simulink library "newTires"  (R2019b)
settings: Solver=ode45  StartTime=0.0  StopTime=10.0  RelTol=1e-3  EnableMultiTasking=on
libraries: vehdynlibtirecommon x6, autolibshared x4, autolibsharedcommon x1
(part 3 of 3)

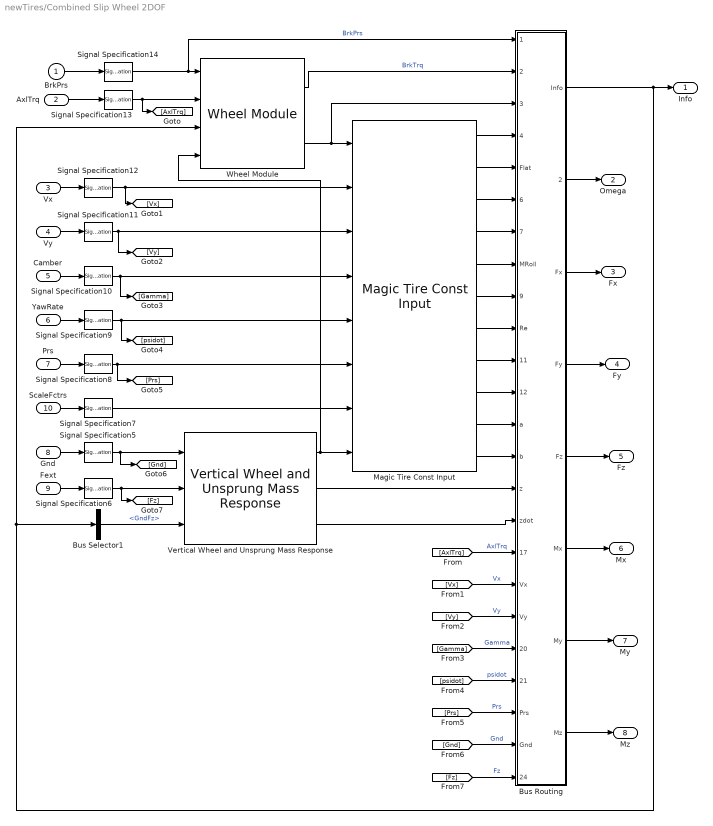
== system newTires/Combined Slip Wheel 2DOF ==
  BrkPrs : Inport
  AxlTrq : Inport  Port=2
  Vx : Inport  Port=3
  Vy : Inport  Port=4
  Camber : Inport  Port=5
  YawRate : Inport  Port=6
  Prs : Inport  Port=7
  Gnd : Inport  Port=8
  Fext : Inport  Port=9
  ScaleFctrs : Inport  Port=10
  Bus Selector1 : BusSelector  OutputSignals=GndFz
  Bus Routing : Subsystem
  Magic Tire Const Input : vehdynlibtirecommon/Magic Tire Const Input  SystemSampleTime=-1  Latency=0  AutoFrameSizeCalculation=off
      settings: SourceProductName=Vehicle Dynamics Blockset  SourceProductBaseCode=VE
  Signal Specification10 : SignalSpecification  Unit=rad
  Signal Specification11 : SignalSpecification  Unit=m/s
  Signal Specification12 : SignalSpecification  Unit=m/s
  Signal Specification13 : SignalSpecification  Unit=N*m
  Signal Specification14 : SignalSpecification  Unit=Pa
  Signal Specification5 : SignalSpecification  Unit=m
  Signal Specification6 : SignalSpecification  Unit=N
  Signal Specification7 : SignalSpecification  Unit=1
  Signal Specification8 : SignalSpecification  Unit=Pa
  Signal Specification9 : SignalSpecification  Unit=rad/s
  Vertical Wheel and Unsprung Mass Response : vehdynlibtirecommon/Vertical Wheel and Unsprung Mass Response  m=MASS  bz=VERTICAL_DAMPING  zo=zo  zdoto=zdoto  g=GRAVITY  ReMax=UNLOADED_RADIUS
      settings: SourceProductName=Vehicle Dynamics Blockset  SourceProductBaseCode=VE
  Wheel Module : vehdynlibtirecommon/Wheel Module  Iyy=IYY
      settings: SourceProductName=Vehicle Dynamics Blockset  SourceProductBaseCode=VE
  Info : Outport  VectorParamsAs1DForOutWhenUnconnected=off
  Omega : Outport  Port=2  Unit=rad/s  VectorParamsAs1DForOutWhenUnconnected=off
  Fx : Outport  Port=3  Unit=N  VectorParamsAs1DForOutWhenUnconnected=off
  Fy : Outport  Port=4  Unit=N  VectorParamsAs1DForOutWhenUnconnected=off
  Fz : Outport  Port=5  Unit=N  VectorParamsAs1DForOutWhenUnconnected=off
  Mx : Outport  Port=6  Unit=N*m  VectorParamsAs1DForOutWhenUnconnected=off
  My : Outport  Port=7  Unit=N*m  VectorParamsAs1DForOutWhenUnconnected=off
  Mz : Outport  Port=8  Unit=N*m  VectorParamsAs1DForOutWhenUnconnected=off
  wires:
  Wheel Module/1 -> Bus Routing/2(BrkTrq)  "BrkTrq"
  Vertical Wheel and Unsprung Mass Response/1 -> Magic Tire Const Input/8, Wheel Module/4
  Wheel Module/2 -> Magic Tire Const Input/1, Bus Routing/3(omega)
  Signal Specification5/1 -> [Gnd], Vertical Wheel and Unsprung Mass Response/1
  Gnd/1 -> Signal Specification5/1
  Fext/1 -> Signal Specification6/1
  Signal Specification6/1 -> [Fz], Vertical Wheel and Unsprung Mass Response/2
  Signal Specification7/1 -> Magic Tire Const Input/7
  Prs/1 -> Signal Specification8/1
  Signal Specification8/1 -> [Prs], Magic Tire Const Input/6
  YawRate/1 -> Signal Specification9/1
  Signal Specification9/1 -> [psidot], Magic Tire Const Input/5
  ScaleFctrs/1 -> Signal Specification7/1
  Signal Specification10/1 -> [Gamma], Magic Tire Const Input/4
  Camber/1 -> Signal Specification10/1
  Signal Specification11/1 -> [Vy], Magic Tire Const Input/3
  Vy/1 -> Signal Specification11/1
  Vx/1 -> Signal Specification12/1
  Signal Specification12/1 -> [Vx], Magic Tire Const Input/2
  Signal Specification13/1 -> [AxlTrq], Wheel Module/2
  AxlTrq/1 -> Signal Specification13/1
  Signal Specification14/1 -> Bus Routing/1(BrkPrs), Wheel Module/1  "BrkPrs"
  Bus Selector1/1 -> Vertical Wheel and Unsprung Mass Response/3  "<GndFz>"
  BrkPrs/1 -> Signal Specification14/1
  Bus Routing/1(Info) -> Bus Selector1/1, Wheel Module/3, Info/1
  Magic Tire Const Input/1 -> Bus Routing/4(FLong)
  Magic Tire Const Input/2 -> Bus Routing/5(Flat)
  Magic Tire Const Input/3 -> Bus Routing/6(FzTire)
  Magic Tire Const Input/4 -> Bus Routing/7(MOver)
  Magic Tire Const Input/5 -> Bus Routing/8(MRoll)
  Magic Tire Const Input/6 -> Bus Routing/9(MAlign)
  Magic Tire Const Input/7 -> Bus Routing/10(Re)
  Magic Tire Const Input/8 -> Bus Routing/11(Kappa)
  Magic Tire Const Input/9 -> Bus Routing/12(Alpha)
  Magic Tire Const Input/10 -> Bus Routing/13(a)
  Magic Tire Const Input/11 -> Bus Routing/14(b)
  Vertical Wheel and Unsprung Mass Response/2 -> Bus Routing/15(z)
  Vertical Wheel and Unsprung Mass Response/3 -> Bus Routing/16(zdot)
  Bus Routing/2(Omega) -> Omega/1
  Bus Routing/3(Fx) -> Fx/1
  Bus Routing/4(Fy) -> Fy/1
  Bus Routing/5(Fz) -> Fz/1
  Bus Routing/6(Mx) -> Mx/1
  Bus Routing/7(My) -> My/1
  Bus Routing/8(Mz) -> Mz/1
  [AxlTrq] -> Bus Routing/17(AxlTrq)  "AxlTrq"
  [Vx] -> Bus Routing/18(Vx)  "Vx"
  [Vy] -> Bus Routing/19(Vy)  "Vy"
  [Gamma] -> Bus Routing/20(Gamma)  "Gamma"
  [psidot] -> Bus Routing/21(psidot)  "psidot"
  [Prs] -> Bus Routing/22(Prs)  "Prs"
  [Gnd] -> Bus Routing/23(Gnd)  "Gnd"
  [Fz] -> Bus Routing/24(FNormal)  "Fz"

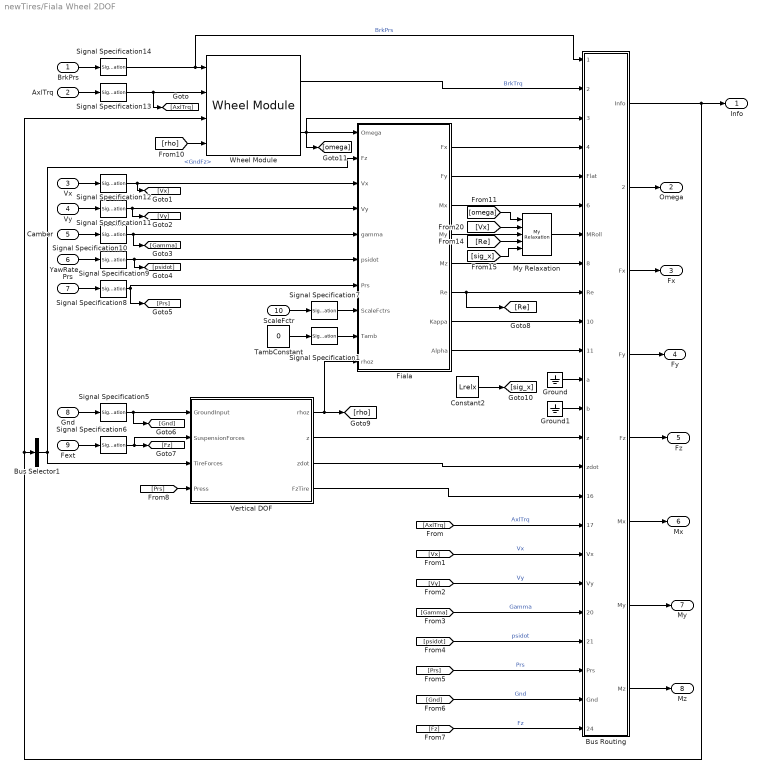
== system newTires/Fiala Wheel 2DOF ==
  BrkPrs : Inport
  AxlTrq : Inport  Port=2
  Vx : Inport  Port=3
  Vy : Inport  Port=4
  Camber : Inport  Port=5
  YawRate : Inport  Port=6
  Prs : Inport  Port=7
  Gnd : Inport  Port=8
  Fext : Inport  Port=9  Unit=N
  ScaleFctr : Inport  Port=10
  Bus Selector1 : BusSelector  OutputSignals=GndFz
  Bus Routing : Subsystem
  Constant2 : Constant  Value=Lrelx
  Fiala : Subsystem
  Ground : Ground
  Ground1 : Ground
  My Relaxation : vehdynlibtirecommon/Magic Tire Const Input/My Relaxation  UpperValue=.001
      settings: SourceProductName=Vehicle Dynamics Blockset  SourceProductBaseCode=VE
  Signal Specification1 : SignalSpecification  Unit=K
  Signal Specification10 : SignalSpecification  Unit=rad
  Signal Specification11 : SignalSpecification  Unit=m/s
  Signal Specification12 : SignalSpecification  Unit=m/s
  Signal Specification13 : SignalSpecification  Unit=N*m
  Signal Specification14 : SignalSpecification  Unit=Pa
  Signal Specification5 : SignalSpecification  Unit=m
  Signal Specification6 : SignalSpecification  Unit=N
  Signal Specification7 : SignalSpecification  Unit=1
  Signal Specification8 : SignalSpecification  Unit=Pa
  Signal Specification9 : SignalSpecification  Unit=rad/s
  TambConstant : Constant  Value=0
  Vertical DOF : Subsystem  VariantControlMode=Label  Variant=on  VariantControl=Variant1  LabelModeActiveChoice=None
  Wheel Module : vehdynlibtirecommon/Wheel Module  Iyy=IYY
      settings: SourceProductName=Vehicle Dynamics Blockset  SourceProductBaseCode=VE
  Info : Outport  VectorParamsAs1DForOutWhenUnconnected=off
  Omega : Outport  Port=2  Unit=rad/s  VectorParamsAs1DForOutWhenUnconnected=off
  Fx : Outport  Port=3  Unit=N  VectorParamsAs1DForOutWhenUnconnected=off
  Fy : Outport  Port=4  Unit=N  VectorParamsAs1DForOutWhenUnconnected=off
  Fz : Outport  Port=5  Unit=N  VectorParamsAs1DForOutWhenUnconnected=off
  Mx : Outport  Port=6  Unit=N*m  VectorParamsAs1DForOutWhenUnconnected=off
  My : Outport  Port=7  Unit=N*m  VectorParamsAs1DForOutWhenUnconnected=off
  Mz : Outport  Port=8  Unit=N*m  VectorParamsAs1DForOutWhenUnconnected=off
  wires:
  Constant2/1 -> [sig_x]
  Fiala/6(Re) -> [Re], Bus Routing/9(Re)
  [Re] -> My Relaxation/4
  [omega] -> My Relaxation/1
  [Vx] -> My Relaxation/2
  [sig_x] -> My Relaxation/5
  Wheel Module/1 -> Bus Routing/2(BrkTrq)  "BrkTrq"
  Wheel Module/2 -> Fiala/1(Omega), Bus Routing/3(omega), [omega]
  Signal Specification5/1 -> [Gnd], Vertical DOF/1("GroundInput ")
  Gnd/1 -> Signal Specification5/1
  Fext/1 -> Signal Specification6/1
  Signal Specification6/1 -> [Fz], Vertical DOF/2("SuspensionForces ")
  Signal Specification7/1 -> Fiala/8(ScaleFctrs)
  Prs/1 -> Signal Specification8/1
  Signal Specification8/1 -> Fiala/7(Prs), [Prs]
  YawRate/1 -> Signal Specification9/1
  Signal Specification9/1 -> Fiala/6(psidot), [psidot]
  ScaleFctr/1 -> Signal Specification7/1
  Signal Specification10/1 -> Fiala/5(gamma), [Gamma]
  Camber/1 -> Signal Specification10/1
  Signal Specification11/1 -> [Vy], Fiala/4(Vy)
  Vy/1 -> Signal Specification11/1
  Vx/1 -> Signal Specification12/1
  Signal Specification12/1 -> [Vx], Fiala/3(Vx)
  Signal Specification13/1 -> [AxlTrq], Wheel Module/2
  AxlTrq/1 -> Signal Specification13/1
  Signal Specification14/1 -> Bus Routing/1(BrkPrs), Wheel Module/1  "BrkPrs"
  Bus Selector1/1 -> Fiala/2(Fz), Vertical DOF/3("TireForces ")  "<GndFz>"
  Bus Routing/1(Info) -> Bus Selector1/1, Wheel Module/3, Info/1
  Fiala/5(Mz) -> Bus Routing/8(MAlign)
  Fiala/7(Kappa) -> Bus Routing/10(Kappa)
  Fiala/8(Alpha) -> Bus Routing/11(Alpha)
  Ground/1 -> Bus Routing/12(a)
  Ground1/1 -> Bus Routing/13(b)
  Bus Routing/2(Omega) -> Omega/1
  Bus Routing/3(Fx) -> Fx/1
  Bus Routing/4(Fy) -> Fy/1
  Bus Routing/5(Fz) -> Fz/1
  Bus Routing/6(Mx) -> Mx/1
  Bus Routing/7(My) -> My/1
  Bus Routing/8(Mz) -> Mz/1
  [AxlTrq] -> Bus Routing/17(AxlTrq)  "AxlTrq"
  [Vx] -> Bus Routing/18(Vx)  "Vx"
  [Vy] -> Bus Routing/19(Vy)  "Vy"
  [Gamma] -> Bus Routing/20(Gamma)  "Gamma"
  [psidot] -> Bus Routing/21(psidot)  "psidot"
  [Prs] -> Bus Routing/22(Prs)  "Prs"
  [Gnd] -> Bus Routing/23(Gnd)  "Gnd"
  [Fz] -> Bus Routing/24(FNormal)  "Fz"
  Fiala/3(Mx) -> Bus Routing/6(MOver)
  Fiala/2(Fy) -> Bus Routing/5(Flat)
  Fiala/1(Fx) -> Bus Routing/4(FLong)
  Fiala/4(My) -> My Relaxation/3
  My Relaxation/1 -> Bus Routing/7(MRoll)
  [rho] -> Wheel Module/4
  BrkPrs/1 -> Signal Specification14/1
  Signal Specification1/1 -> Fiala/9(Tamb)
  Vertical DOF/1(" rhoz") -> Fiala/10(rhoz), [rho]
  Vertical DOF/2(" z") -> Bus Routing/14(z)
  Vertical DOF/3(" zdot") -> Bus Routing/15(zdot)
  [Prs] -> Vertical DOF/4(Press)
  TambConstant/1 -> Signal Specification1/1
  Vertical DOF/4(FzTire) -> Bus Routing/16(GndFz)

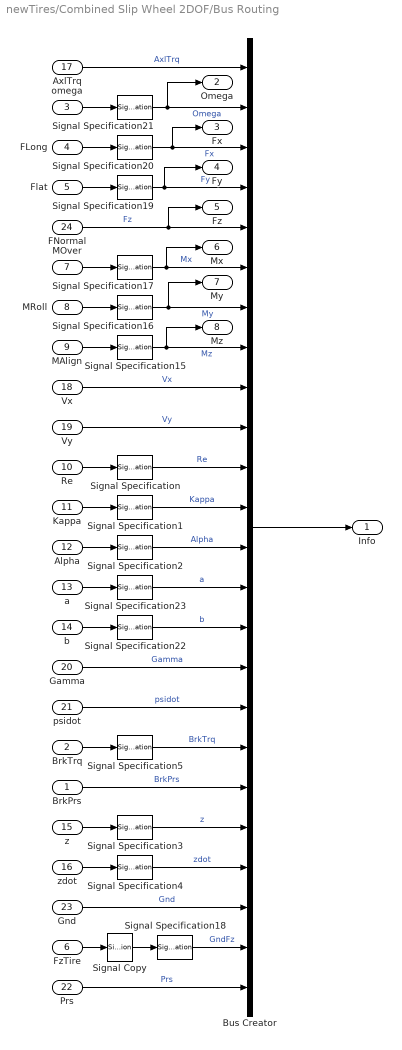
== system newTires/Combined Slip Wheel 2DOF/Bus Routing ==
  BrkPrs : Inport
  BrkTrq : Inport  Port=2
  omega : Inport  Port=3
  FLong : Inport  Port=4
  Flat : Inport  Port=5
  FzTire : Inport  Port=6
  MOver : Inport  Port=7
  MRoll : Inport  Port=8
  MAlign : Inport  Port=9
  Re : Inport  Port=10
  Kappa : Inport  Port=11
  Alpha : Inport  Port=12
  a : Inport  Port=13
  b : Inport  Port=14
  z : Inport  Port=15
  zdot : Inport  Port=16
  AxlTrq : Inport  Port=17
  Vx : Inport  Port=18
  Vy : Inport  Port=19
  Gamma : Inport  Port=20
  psidot : Inport  Port=21
  Prs : Inport  Port=22
  Gnd : Inport  Port=23
  FNormal : Inport  Port=24
  Bus Creator : BusCreator  Inputs=24
  Signal Copy : SignalConversion  OverrideOpt=off
  Signal Specification{,3,22..23} (4 alike) : SignalSpecification  Unit=m
  Signal Specification1 : SignalSpecification  Unit=1
  Signal Specification{5,15..17} (4 alike) : SignalSpecification  Unit=N*m
  Signal Specification18 : SignalSpecification  Unit=N
  Signal Specification19 : SignalSpecification  Unit=N
  Signal Specification2 : SignalSpecification  Unit=rad
  Signal Specification20 : SignalSpecification  Unit=N
  Signal Specification21 : SignalSpecification  Unit=rad/s
  Signal Specification4 : SignalSpecification  Unit=m/s
  Info : Outport  VectorParamsAs1DForOutWhenUnconnected=off
  Omega : Outport  Port=2  Unit=rad/s  VectorParamsAs1DForOutWhenUnconnected=off
  Fx : Outport  Port=3  Unit=N  VectorParamsAs1DForOutWhenUnconnected=off
  Fy : Outport  Port=4  Unit=N  VectorParamsAs1DForOutWhenUnconnected=off
  Fz : Outport  Port=5  Unit=N  VectorParamsAs1DForOutWhenUnconnected=off
  Mx : Outport  Port=6  Unit=N*m  VectorParamsAs1DForOutWhenUnconnected=off
  My : Outport  Port=7  Unit=N*m  VectorParamsAs1DForOutWhenUnconnected=off
  Mz : Outport  Port=8  Unit=N*m  VectorParamsAs1DForOutWhenUnconnected=off
  wires:
  Signal Specification3/1 -> Bus Creator/20  "z"
  a/1 -> Signal Specification23/1
  Alpha/1 -> Signal Specification2/1
  Signal Specification4/1 -> Bus Creator/21  "zdot"
  Signal Specification21/1 -> Bus Creator/2, Omega/1  "Omega"
  FNormal/1 -> Bus Creator/5, Fz/1  "Fz"
  Signal Specification15/1 -> Bus Creator/8, Mz/1  "Mz"
  Signal Specification/1 -> Bus Creator/11  "Re"
  Bus Creator/1 -> Info/1
  Signal Specification17/1 -> Mx/1, Bus Creator/6  "Mx"
  MOver/1 -> Signal Specification17/1
  Signal Specification1/1 -> Bus Creator/12  "Kappa"
  FLong/1 -> Signal Specification20/1
  Signal Specification19/1 -> Bus Creator/4, Fy/1  "Fy"
  Signal Specification16/1 -> Bus Creator/7, My/1  "My"
  omega/1 -> Signal Specification21/1
  Signal Specification2/1 -> Bus Creator/13  "Alpha"
  Signal Specification20/1 -> Bus Creator/3, Fx/1  "Fx"
  Signal Specification23/1 -> Bus Creator/14  "a"
  Signal Specification22/1 -> Bus Creator/15  "b"
  FzTire/1 -> Signal Copy/1
  MAlign/1 -> Signal Specification15/1
  Flat/1 -> Signal Specification19/1
  b/1 -> Signal Specification22/1
  Re/1 -> Signal Specification/1
  zdot/1 -> Signal Specification4/1
  z/1 -> Signal Specification3/1
  MRoll/1 -> Signal Specification16/1
  Kappa/1 -> Signal Specification1/1
  BrkTrq/1 -> Signal Specification5/1
  AxlTrq/1 -> Bus Creator/1  "AxlTrq"
  Vx/1 -> Bus Creator/9  "Vx"
  Vy/1 -> Bus Creator/10  "Vy"
  Gamma/1 -> Bus Creator/16  "Gamma"
  psidot/1 -> Bus Creator/17  "psidot"
  Signal Specification5/1 -> Bus Creator/18  "BrkTrq"
  BrkPrs/1 -> Bus Creator/19  "BrkPrs"
  Signal Specification18/1 -> Bus Creator/23  "GndFz"
  Gnd/1 -> Bus Creator/22  "Gnd"
  Prs/1 -> Bus Creator/24  "Prs"
  Signal Copy/1 -> Signal Specification18/1

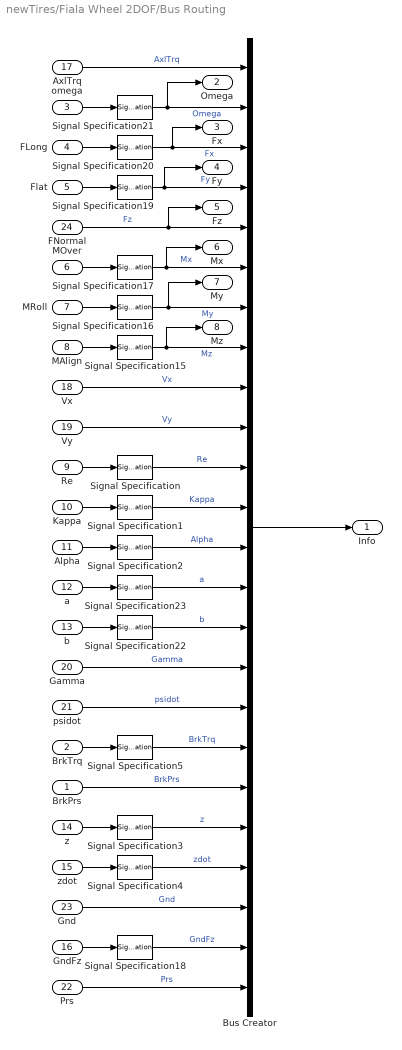
== system newTires/Fiala Wheel 2DOF/Bus Routing ==
  BrkPrs : Inport
  BrkTrq : Inport  Port=2
  omega : Inport  Port=3
  FLong : Inport  Port=4
  Flat : Inport  Port=5
  MOver : Inport  Port=6
  MRoll : Inport  Port=7
  MAlign : Inport  Port=8
  Re : Inport  Port=9
  Kappa : Inport  Port=10
  Alpha : Inport  Port=11
  a : Inport  Port=12
  b : Inport  Port=13
  z : Inport  Port=14
  zdot : Inport  Port=15
  GndFz : Inport  Port=16
  AxlTrq : Inport  Port=17
  Vx : Inport  Port=18
  Vy : Inport  Port=19
  Gamma : Inport  Port=20
  psidot : Inport  Port=21
  Prs : Inport  Port=22
  Gnd : Inport  Port=23
  FNormal : Inport  Port=24
  Bus Creator : BusCreator  Inputs=24
  Signal Specification{,3,22..23} (4 alike) : SignalSpecification  Unit=m
  Signal Specification1 : SignalSpecification  Unit=1
  Signal Specification{5,15..17} (4 alike) : SignalSpecification  Unit=N*m
  Signal Specification18 : SignalSpecification  Unit=N
  Signal Specification19 : SignalSpecification  Unit=N
  Signal Specification2 : SignalSpecification  Unit=rad
  Signal Specification20 : SignalSpecification  Unit=N
  Signal Specification21 : SignalSpecification  Unit=rad/s
  Signal Specification4 : SignalSpecification  Unit=m/s
  Info : Outport  VectorParamsAs1DForOutWhenUnconnected=off
  Omega : Outport  Port=2  Unit=rad/s  VectorParamsAs1DForOutWhenUnconnected=off
  Fx : Outport  Port=3  Unit=N  VectorParamsAs1DForOutWhenUnconnected=off
  Fy : Outport  Port=4  Unit=N  VectorParamsAs1DForOutWhenUnconnected=off
  Fz : Outport  Port=5  Unit=N  VectorParamsAs1DForOutWhenUnconnected=off
  Mx : Outport  Port=6  Unit=N*m  VectorParamsAs1DForOutWhenUnconnected=off
  My : Outport  Port=7  Unit=N*m  VectorParamsAs1DForOutWhenUnconnected=off
  Mz : Outport  Port=8  Unit=N*m  VectorParamsAs1DForOutWhenUnconnected=off
  wires:
  Signal Specification3/1 -> Bus Creator/20  "z"
  a/1 -> Signal Specification23/1
  Alpha/1 -> Signal Specification2/1
  Signal Specification4/1 -> Bus Creator/21  "zdot"
  Signal Specification21/1 -> Bus Creator/2, Omega/1  "Omega"
  FNormal/1 -> Bus Creator/5, Fz/1  "Fz"
  Signal Specification15/1 -> Bus Creator/8, Mz/1  "Mz"
  Signal Specification/1 -> Bus Creator/11  "Re"
  Bus Creator/1 -> Info/1
  Signal Specification17/1 -> Mx/1, Bus Creator/6  "Mx"
  MOver/1 -> Signal Specification17/1
  Signal Specification1/1 -> Bus Creator/12  "Kappa"
  FLong/1 -> Signal Specification20/1
  Signal Specification19/1 -> Bus Creator/4, Fy/1  "Fy"
  Signal Specification16/1 -> Bus Creator/7, My/1  "My"
  omega/1 -> Signal Specification21/1
  Signal Specification2/1 -> Bus Creator/13  "Alpha"
  Signal Specification20/1 -> Bus Creator/3, Fx/1  "Fx"
  Signal Specification23/1 -> Bus Creator/14  "a"
  Signal Specification22/1 -> Bus Creator/15  "b"
  GndFz/1 -> Signal Specification18/1
  MAlign/1 -> Signal Specification15/1
  Flat/1 -> Signal Specification19/1
  b/1 -> Signal Specification22/1
  Re/1 -> Signal Specification/1
  zdot/1 -> Signal Specification4/1
  z/1 -> Signal Specification3/1
  MRoll/1 -> Signal Specification16/1
  Kappa/1 -> Signal Specification1/1
  BrkTrq/1 -> Signal Specification5/1
  AxlTrq/1 -> Bus Creator/1  "AxlTrq"
  Vx/1 -> Bus Creator/9  "Vx"
  Vy/1 -> Bus Creator/10  "Vy"
  Gamma/1 -> Bus Creator/16  "Gamma"
  psidot/1 -> Bus Creator/17  "psidot"
  Signal Specification5/1 -> Bus Creator/18  "BrkTrq"
  BrkPrs/1 -> Bus Creator/19  "BrkPrs"
  Signal Specification18/1 -> Bus Creator/23  "GndFz"
  Gnd/1 -> Bus Creator/22  "Gnd"
  Prs/1 -> Bus Creator/24  "Prs"

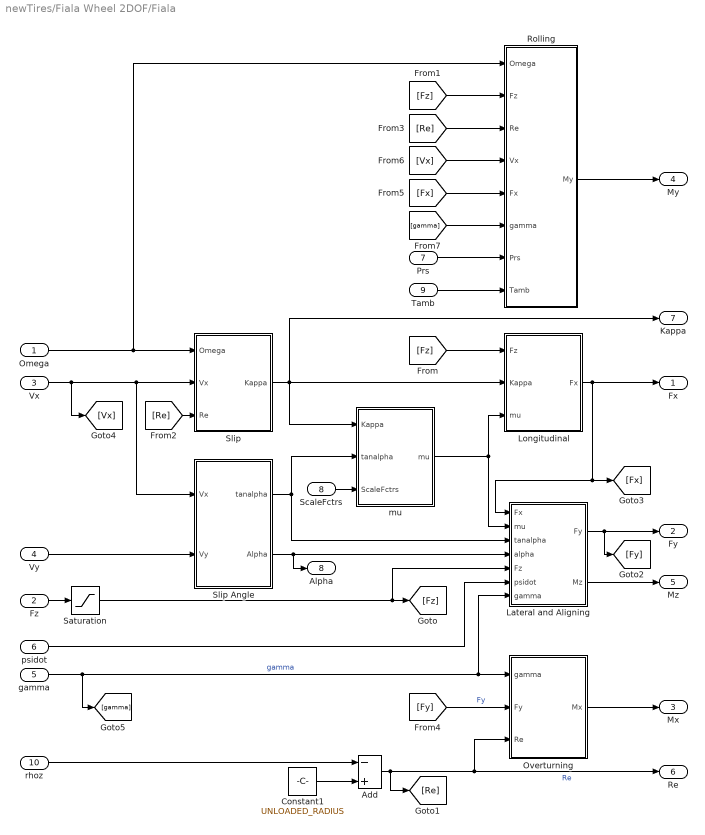
== system newTires/Fiala Wheel 2DOF/Fiala ==
  Omega : Inport
  Fz : Inport  Port=2
  Vx : Inport  Port=3
  Vy : Inport  Port=4
  gamma : Inport  Port=5
  psidot : Inport  Port=6
  Prs : Inport  Port=7
  ScaleFctrs : Inport  Port=8
  Tamb : Inport  Port=9
  rhoz : Inport  Port=10
  Add : Sum  Inputs=-+
  Constant1 : Constant  Value=UNLOADED_RADIUS
  Lateral and Aligning : Subsystem
  Longitudinal : Subsystem
  Overturning : Subsystem
  Rolling : Subsystem  VariantControlMode=Label  Variant=on  VariantControl=Variant1  LabelModeActiveChoice=Simple
  Saturation : Saturate  UpperLimit=FZMAX  LowerLimit=FZMIN  ZeroCross=off
  Slip : Subsystem
  Slip Angle : Subsystem
  mu : Subsystem
  Fx : Outport  VectorParamsAs1DForOutWhenUnconnected=off
  Fy : Outport  Port=2  VectorParamsAs1DForOutWhenUnconnected=off
  Mx : Outport  Port=3  VectorParamsAs1DForOutWhenUnconnected=off
  My : Outport  Port=4  VectorParamsAs1DForOutWhenUnconnected=off
  Mz : Outport  Port=5  VectorParamsAs1DForOutWhenUnconnected=off
  Re : Outport  Port=6  VectorParamsAs1DForOutWhenUnconnected=off
  Kappa : Outport  Port=7  VectorParamsAs1DForOutWhenUnconnected=off
  Alpha : Outport  Port=8  VectorParamsAs1DForOutWhenUnconnected=off
  wires:
  Slip Angle/1(tanalpha) -> mu/2(tanalpha), Lateral and Aligning/3(tanalpha)
  Longitudinal/1(Fx) -> Fx/1, [Fx], Lateral and Aligning/1(Fx)
  Vx/1 -> [Vx], Slip Angle/1(Vx), Slip/2(Vx)
  Lateral and Aligning/2(Mz) -> Mz/1
  Fz/1 -> Saturation/1
  Saturation/1 -> [Fz], Lateral and Aligning/5(Fz)
  mu/1(mu) -> Lateral and Aligning/2(mu), Longitudinal/3(mu)
  Slip/1(Kappa) -> Kappa/1, Longitudinal/2(Kappa), mu/1(Kappa)
  Lateral and Aligning/1(Fy) -> [Fy], Fy/1
  Omega/1 -> Slip/1(Omega), Rolling/1("Omega ")
  [Fz] -> Longitudinal/1(Fz)
  Vy/1 -> Slip Angle/2(Vy)
  Slip Angle/2(Alpha) -> Alpha/1, Lateral and Aligning/4(alpha)
  Constant1/1 -> Add/2
  rhoz/1 -> Add/1
  Add/1 -> Re/1, Overturning/3(Re), [Re]  "Re"
  psidot/1 -> Lateral and Aligning/6(psidot)
  ScaleFctrs/1 -> mu/3(ScaleFctrs)
  gamma/1 -> [gamma], Lateral and Aligning/7(gamma), Overturning/1(gamma)  "gamma"
  [Re] -> Slip/3(Re)
  [Fy] -> Overturning/2(Fy)  "Fy"
  Overturning/1(Mx) -> Mx/1
  Prs/1 -> Rolling/7(Prs)
  [Fz] -> Rolling/2("Fz ")
  [Re] -> Rolling/3(Re)
  Rolling/1(" My") -> My/1
  [Fx] -> Rolling/5(Fx)
  [Vx] -> Rolling/4(Vx)
  Tamb/1 -> Rolling/8(Tamb)
  [gamma] -> Rolling/6(gamma)

== system newTires/Fiala Wheel 2DOF/Vertical DOF ==
  "GroundInput " : Inport
  "SuspensionForces " : Inport  Port=2
  "TireForces " : Inport  Port=3
  Press : Inport  Port=4
  Mapped Vertical DOF : Subsystem  VariantControl=Mapped
  None : Subsystem  VariantControl=None
  Vertical Wheel and Unsprung Mass Response : vehdynlibtirecommon/Vertical Wheel and Unsprung Mass Response  VariantControl=Linear  m=MASS  bz=VERTICAL_DAMPING  zo=zo  zdoto=zdoto  g=GRAVITY  ReMax=UNLOADED_RADIUS
      settings: SourceProductName=Vehicle Dynamics Blockset  SourceProductBaseCode=VE
  " rhoz" : Outport  VectorParamsAs1DForOutWhenUnconnected=off
  " z" : Outport  Port=2  VectorParamsAs1DForOutWhenUnconnected=off
  " zdot" : Outport  Port=3  VectorParamsAs1DForOutWhenUnconnected=off
  FzTire : Outport  Port=4  VectorParamsAs1DForOutWhenUnconnected=off

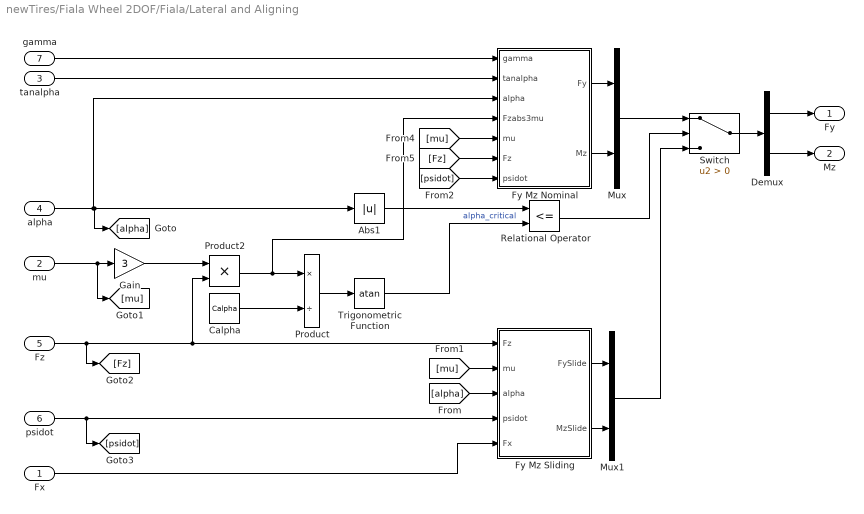
== system newTires/Fiala Wheel 2DOF/Fiala/Lateral and Aligning ==
  Fx : Inport
  mu : Inport  Port=2
  tanalpha : Inport  Port=3
  alpha : Inport  Port=4
  Fz : Inport  Port=5
  psidot : Inport  Port=6
  gamma : Inport  Port=7
  Abs1 : Abs  ZeroCross=off
  Calpha : Constant  Value=Calpha
  Demux : Demux  Outputs=2
  Fy Mz Nominal : Subsystem
  Fy Mz Sliding : Subsystem
  Gain : Gain  Gain=3
  Mux : Mux  Inputs=2
  Mux1 : Mux  Inputs=2
  Product : Product  Inputs=*/
  Product2 : Product
  Relational Operator : RelationalOperator  Operator=<=  OutDataTypeStr=boolean  RndMeth=Simplest
  Switch : Switch  Criteria=u2 > Threshold
  Trigonometric Function : Trigonometry  Operator=atan
  Fy : Outport  VectorParamsAs1DForOutWhenUnconnected=off
  Mz : Outport  Port=2  VectorParamsAs1DForOutWhenUnconnected=off
  wires:
  [mu] -> Fy Mz Sliding/2(mu)
  [alpha] -> Fy Mz Sliding/3(alpha)
  Fy Mz Sliding/1(FySlide) -> Mux1/1
  mu/1 -> Gain/1, [mu]
  Switch/1 -> Demux/1
  Relational Operator/1 -> Switch/2
  Calpha/1 -> Product/2
  Trigonometric Function/1 -> Relational Operator/2  "alpha_critical"
  Product/1 -> Trigonometric Function/1
  Abs1/1 -> Relational Operator/1
  Gain/1 -> Product2/1
  Product2/1 -> Fy Mz Nominal/4(Fzabs3mu), Product/1
  tanalpha/1 -> Fy Mz Nominal/2(tanalpha)
  [mu] -> Fy Mz Nominal/5(mu)
  alpha/1 -> Abs1/1, [alpha], Fy Mz Nominal/3(alpha)
  [Fz] -> Fy Mz Nominal/6(Fz)
  Fy Mz Nominal/1(Fy) -> Mux/1
  Fy Mz Nominal/2(Mz) -> Mux/2
  Mux/1 -> Switch/1
  Demux/1 -> Fy/1
  Demux/2 -> Mz/1
  Fy Mz Sliding/2(MzSlide) -> Mux1/2
  Mux1/1 -> Switch/3
  Fz/1 -> Product2/2, Fy Mz Sliding/1(Fz), [Fz]
  psidot/1 -> [psidot], Fy Mz Sliding/4(psidot)
  [psidot] -> Fy Mz Nominal/7(psidot)
  gamma/1 -> Fy Mz Nominal/1(gamma)
  Fx/1 -> Fy Mz Sliding/5(Fx)

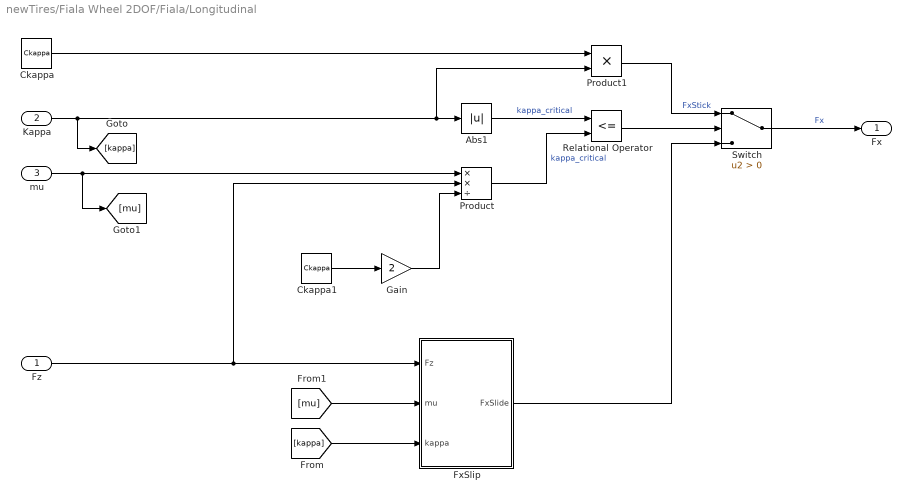
== system newTires/Fiala Wheel 2DOF/Fiala/Longitudinal ==
  Fz : Inport
  Kappa : Inport  Port=2
  mu : Inport  Port=3
  Abs1 : Abs  ZeroCross=off
  Ckappa : Constant  Value=Ckappa
  Ckappa1 : Constant  Value=Ckappa
  FxSlip : Subsystem
  Gain : Gain  Gain=2
  Product : Product  Inputs=**/
  Product1 : Product
  Relational Operator : RelationalOperator  Operator=<=  OutDataTypeStr=boolean  RndMeth=Simplest
  Switch : Switch  Criteria=u2 > Threshold
  Fx : Outport  VectorParamsAs1DForOutWhenUnconnected=off
  wires:
  Ckappa/1 -> Product1/1
  Kappa/1 -> [kappa], Abs1/1, Product1/2
  Gain/1 -> Product/3
  Product/1 -> Relational Operator/2  "kappa_critical"
  Product1/1 -> Switch/1  "FxStick"
  Relational Operator/1 -> Switch/2
  Switch/1 -> Fx/1  "Fx"
  mu/1 -> [mu], Product/1
  Fz/1 -> Product/2, FxSlip/1(Fz)
  FxSlip/1(FxSlide) -> Switch/3
  [kappa] -> FxSlip/3(kappa)
  [mu] -> FxSlip/2(mu)
  Abs1/1 -> Relational Operator/1  "kappa_critical"
  Ckappa1/1 -> Gain/1

== system newTires/Fiala Wheel 2DOF/Fiala/Overturning ==
  gamma : Inport
  Fy : Inport  Port=2
  Re : Inport  Port=3
  Product : Product  Inputs=3
  Trigonometric Function : Trigonometry  Operator=cos
  Mx : Outport  VectorParamsAs1DForOutWhenUnconnected=off
  wires:
  Trigonometric Function/1 -> Product/1
  Re/1 -> Product/3
  Product/1 -> Mx/1  "Mx"
  Fy/1 -> Product/2
  gamma/1 -> Trigonometric Function/1

== system newTires/Fiala Wheel 2DOF/Fiala/Rolling ==
  "Omega " : Inport
  "Fz " : Inport  Port=2
  Re : Inport  Port=3
  Vx : Inport  Port=4
  Fx : Inport  Port=5
  gamma : Inport  Port=6
  Prs : Inport  Port=7
  Tamb : Inport  Port=8
  ISO : Subsystem  VariantControl=ISO
  MagicFormula : Subsystem  VariantControl=MagicFormula
  Mapped : Subsystem  VariantControl=Mapped
  None : Subsystem  VariantControl=None
  Simple : Subsystem  VariantControl=Simple
  " My" : Outport  VectorParamsAs1DForOutWhenUnconnected=off

== system newTires/Fiala Wheel 2DOF/Fiala/Slip ==
  Omega : Inport
  Vx : Inport  Port=2
  Re : Inport  Port=3
  1/Lrelx : Gain  Gain=1/Lrelx
  Abs : Abs  ZeroCross=off
  Integrator : Integrator
  Product : Product
  Product2 : Product
  Subtract : Sum  Inputs=+--
  Kappa : Outport  VectorParamsAs1DForOutWhenUnconnected=off
  wires:
  1/Lrelx/1 -> Kappa/1, Product2/2
  Subtract/1 -> Integrator/1
  Product/1 -> Subtract/1  "Vsx"
  Abs/1 -> Product2/1
  Re/1 -> Product/1
  Product2/1 -> Subtract/3  "Vsx'"
  Vx/1 -> Subtract/2, Abs/1
  Integrator/1 -> 1/Lrelx/1  "u"
  Omega/1 -> Product/2

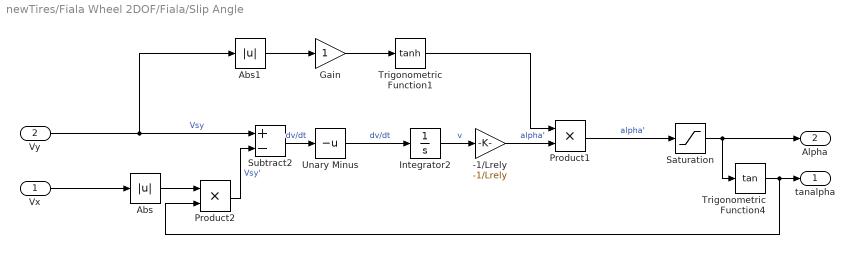
== system newTires/Fiala Wheel 2DOF/Fiala/Slip Angle ==
  Vx : Inport
  Vy : Inport  Port=2
  -1/Lrely : Gain  Gain=-1/Lrely
  Abs : Abs  ZeroCross=off
  Abs1 : Abs  ZeroCross=off
  Gain : Gain
  Integrator2 : Integrator
  Product1 : Product
  Product2 : Product
  Saturation : Saturate  UpperLimit=ALPMAX  LowerLimit=ALPMIN  ZeroCross=off
  Subtract2 : Sum  Inputs=+-
  Trigonometric Function1 : Trigonometry  Operator=tanh
  Trigonometric Function4 : Trigonometry  Operator=tan
  Unary Minus : UnaryMinus
  tanalpha : Outport  VectorParamsAs1DForOutWhenUnconnected=off
  Alpha : Outport  Port=2  VectorParamsAs1DForOutWhenUnconnected=off
  wires:
  Vy/1 -> Abs1/1, Subtract2/1  "Vsy"
  Vx/1 -> Abs/1
  Abs/1 -> Product2/1
  Integrator2/1 -> -1/Lrely/1  "v"
  Unary Minus/1 -> Integrator2/1  "dv/dt"
  Subtract2/1 -> Unary Minus/1  "dv/dt"
  Product2/1 -> Subtract2/2  "Vsy'"
  Saturation/1 -> Trigonometric Function4/1, Alpha/1
  Trigonometric Function4/1 -> Product2/2, tanalpha/1
  -1/Lrely/1 -> Product1/2  "alpha'"
  Abs1/1 -> Gain/1
  Gain/1 -> Trigonometric Function1/1
  Product1/1 -> Saturation/1  "alpha'"
  Trigonometric Function1/1 -> Product1/1

== system newTires/Fiala Wheel 2DOF/Fiala/mu ==
  Kappa : Inport
  tanalpha : Inport  Port=2
  ScaleFctrs : Inport  Port=3
  Product{1..2,4..5} (4 alike) : Product
  Saturation : Saturate  UpperLimit=1  LowerLimit=0  ZeroCross=off
  Sqrt : Sqrt  SaturateOnIntegerOverflow=on
  Subtract2 : Sum
  Subtract3 : Sum  Inputs=+-
  Subtract4 : Sum  Inputs=+-
  muMax : Constant  Value=muMax
  muMin : Constant  Value=muMin
  mu : Outport  VectorParamsAs1DForOutWhenUnconnected=off
  wires:
  Subtract2/1 -> Sqrt/1
  muMax/1 -> Subtract3/1, Subtract4/1
  Kappa/1 -> Product5/2, Product5/1
  Saturation/1 -> Product4/2  "KappaAlpha"
  Product4/1 -> Subtract4/2
  Subtract3/1 -> Product4/1
  Product5/1 -> Subtract2/1
  Sqrt/1 -> Saturation/1
  muMin/1 -> Subtract3/2
  tanalpha/1 -> Product1/2, Product1/1
  Product1/1 -> Subtract2/2
  Product2/1 -> mu/1  "mu"
  ScaleFctrs/1 -> Product2/2
  Subtract4/1 -> Product2/1

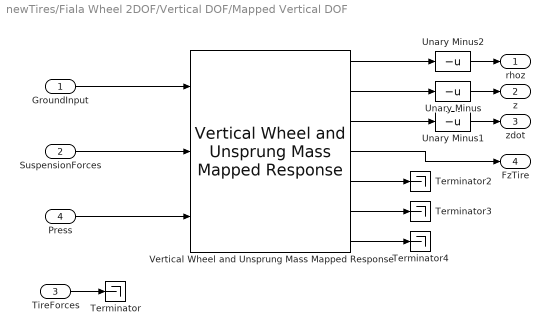
== system newTires/Fiala Wheel 2DOF/Vertical DOF/Mapped Vertical DOF ==
  "GroundInput " : Inport
  "SuspensionForces " : Inport  Port=2
  "TireForces " : Inport  Port=3
  Press : Inport  Port=4
  Terminator{,2..4} (4 alike) : Terminator
  Unary Minus : UnaryMinus
  Unary Minus1 : UnaryMinus
  Unary Minus2 : UnaryMinus
  Vertical Wheel and Unsprung Mass Mapped Response : autolibsharedcommon/Vertical Wheel and Unsprung Mass Mapped Response  m=MASS  zFz=zFz  zdotFz=zdotFz  Fzz=Fzz  pFz=pFz  Fzzdot=Fzzdot  zo=zo  zdoto=zdoto  g=-GRAVITY
      settings: SourceProductName=Powertrain Blockset  SourceProductBaseCode=PW
  rhoz : Outport  VectorParamsAs1DForOutWhenUnconnected=off
  z : Outport  Port=2  VectorParamsAs1DForOutWhenUnconnected=off
  zdot : Outport  Port=3  VectorParamsAs1DForOutWhenUnconnected=off
  FzTire : Outport  Port=4  VectorParamsAs1DForOutWhenUnconnected=off
  wires:
  Press/1 -> Vertical Wheel and Unsprung Mass Mapped Response/3
  Vertical Wheel and Unsprung Mass Mapped Response/4 -> FzTire/1
  "TireForces "/1 -> Terminator/1
  "GroundInput "/1 -> Vertical Wheel and Unsprung Mass Mapped Response/1
  Vertical Wheel and Unsprung Mass Mapped Response/3 -> Unary Minus1/1
  Vertical Wheel and Unsprung Mass Mapped Response/2 -> Unary Minus/1
  Vertical Wheel and Unsprung Mass Mapped Response/1 -> Unary Minus2/1
  "SuspensionForces "/1 -> Vertical Wheel and Unsprung Mass Mapped Response/2
  Vertical Wheel and Unsprung Mass Mapped Response/5 -> Terminator2/1
  Vertical Wheel and Unsprung Mass Mapped Response/7 -> Terminator4/1
  Vertical Wheel and Unsprung Mass Mapped Response/6 -> Terminator3/1
  Unary Minus/1 -> z/1
  Unary Minus1/1 -> zdot/1
  Unary Minus2/1 -> rhoz/1

== system newTires/Fiala Wheel 2DOF/Vertical DOF/None ==
  GroundInput : Inport  PortDimensions=1
  SuspensionForces : Inport  Port=2  PortDimensions=1
  TireForces : Inport  Port=3  PortDimensions=1
  Constant : Constant  Value=0
  Constant1 : Constant  Value=0
  Terminator : Terminator
  rhoz : Outport  VectorParamsAs1DForOutWhenUnconnected=off
  z : Outport  Port=2  VectorParamsAs1DForOutWhenUnconnected=off
  zdot : Outport  Port=3  VectorParamsAs1DForOutWhenUnconnected=off
  FzTire : Outport  Port=4  VectorParamsAs1DForOutWhenUnconnected=off
  wires:
  Constant/1 -> rhoz/1
  TireForces/1 -> Terminator/1
  SuspensionForces/1 -> FzTire/1
  GroundInput/1 -> z/1
  Constant1/1 -> zdot/1

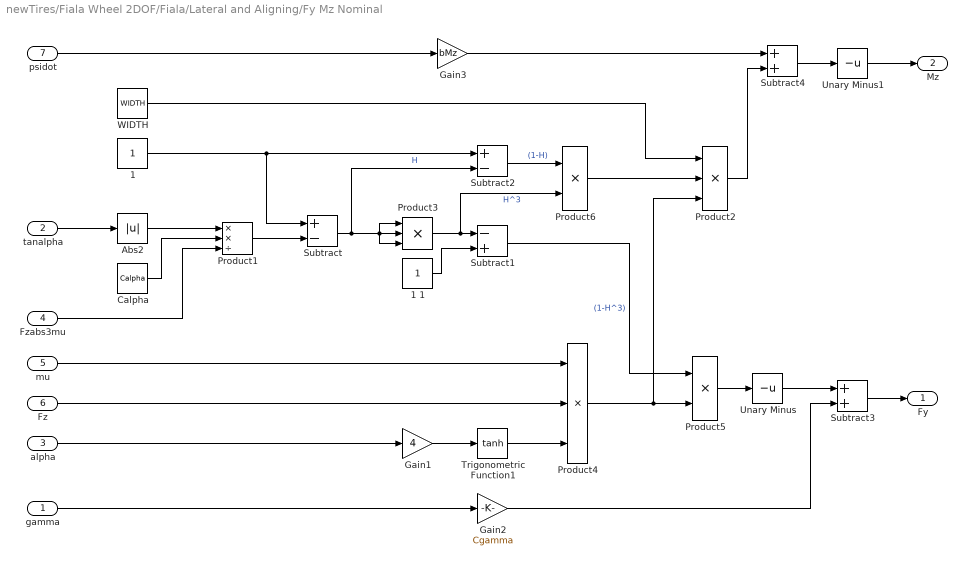
== system newTires/Fiala Wheel 2DOF/Fiala/Lateral and Aligning/Fy Mz Nominal ==
  gamma : Inport
  tanalpha : Inport  Port=2
  alpha : Inport  Port=3
  Fzabs3mu : Inport  Port=4
  mu : Inport  Port=5
  Fz : Inport  Port=6
  psidot : Inport  Port=7
  "1 " : Constant
  1 1 : Constant
  Abs2 : Abs  ZeroCross=off
  Calpha : Constant  Value=Calpha
  Gain1 : Gain  Gain=4
  Gain2 : Gain  Gain=Cgamma
  Gain3 : Gain  Gain=bMz
  Product1 : Product  Inputs=**/
  Product2 : Product  Inputs=***
  Product3 : Product  Inputs=***
  Product4 : Product  Inputs=***
  Product5 : Product  Inputs=**
  Product6 : Product  Inputs=**
  Subtract : Sum  Inputs=+-
  Subtract1 : Sum  Inputs=-+
  Subtract2 : Sum  Inputs=+-
  Subtract3 : Sum
  Subtract4 : Sum
  Trigonometric Function1 : Trigonometry  Operator=tanh
  Unary Minus : UnaryMinus
  Unary Minus1 : UnaryMinus
  WIDTH : Constant  Value=WIDTH
  Fy : Outport  VectorParamsAs1DForOutWhenUnconnected=off
  Mz : Outport  Port=2  VectorParamsAs1DForOutWhenUnconnected=off
  wires:
  Subtract1/1 -> Product5/1  "(1-H^3)"
  Abs2/1 -> Product1/1
  Product1/1 -> Subtract/2
  Subtract/1 -> Subtract2/2, Product3/3, Product3/1, Product3/2  "H"
  Product3/1 -> Product6/2, Subtract1/1  "H^3"
  1 1/1 -> Subtract1/2
  Product4/1 -> Product2/3, Product5/2
  mu/1 -> Product4/1
  Calpha/1 -> Product1/2
  Fz/1 -> Product4/2
  Fzabs3mu/1 -> Product1/3
  tanalpha/1 -> Abs2/1
  Gain1/1 -> Trigonometric Function1/1
  alpha/1 -> Gain1/1
  Trigonometric Function1/1 -> Product4/3
  Product5/1 -> Unary Minus/1
  "1 "/1 -> Subtract/1, Subtract2/1
  Subtract2/1 -> Product6/1  "(1-H)"
  Product6/1 -> Product2/2
  WIDTH/1 -> Product2/1
  psidot/1 -> Gain3/1
  Unary Minus/1 -> Subtract3/1
  gamma/1 -> Gain2/1
  Subtract3/1 -> Fy/1
  Gain2/1 -> Subtract3/2
  Unary Minus1/1 -> Mz/1
  Gain3/1 -> Subtract4/1
  Subtract4/1 -> Unary Minus1/1
  Product2/1 -> Subtract4/2

== system newTires/Fiala Wheel 2DOF/Fiala/Lateral and Aligning/Fy Mz Sliding ==
  Fz : Inport
  mu : Inport  Port=2
  alpha : Inport  Port=3
  psidot : Inport  Port=4
  Fx : Inport  Port=5
  Gain1 : Gain  Gain=4
  Gain3 : Gain  Gain=bMz
  Product2 : Product
  Product4 : Product
  Terminator : Terminator
  Trigonometric Function : Trigonometry  Operator=tanh
  Unary Minus : UnaryMinus
  FySlide : Outport  VectorParamsAs1DForOutWhenUnconnected=off
  MzSlide : Outport  Port=2  VectorParamsAs1DForOutWhenUnconnected=off
  wires:
  Unary Minus/1 -> FySlide/1  "FySlide"
  alpha/1 -> Gain1/1
  mu/1 -> Product2/2
  Trigonometric Function/1 -> Product4/2
  Product2/1 -> Product4/1
  Fz/1 -> Product2/1
  Gain1/1 -> Trigonometric Function/1
  Product4/1 -> Unary Minus/1
  Gain3/1 -> MzSlide/1
  Fx/1 -> Terminator/1
  psidot/1 -> Gain3/1

== system newTires/Fiala Wheel 2DOF/Fiala/Longitudinal/FxSlip ==
  Fz : Inport
  mu : Inport  Port=2
  kappa : Inport  Port=3
  Abs : Abs  ZeroCross=off
  Ckappa : Constant  Value=Ckappa
  Gain1 : Gain  Gain=4
  Product2 : Product
  Product3 : Product  Inputs=**//
  Product4 : Product
  Subtract : Sum  Inputs=+-
  Trigonometric Function : Trigonometry  Operator=tanh
  FxSlide : Outport  VectorParamsAs1DForOutWhenUnconnected=off
  wires:
  Gain1/1 -> Product3/4, Trigonometric Function/1
  Fz/1 -> Product2/1
  Product2/1 -> Subtract/1, Product3/2, Product3/1  "Fx1"
  Subtract/1 -> Product4/1
  Ckappa/1 -> Product3/3
  Trigonometric Function/1 -> Product4/2
  Abs/1 -> Subtract/2  "Fx2"
  mu/1 -> Product2/2
  kappa/1 -> Gain1/1
  Product4/1 -> FxSlide/1  "FxSlide"
  Product3/1 -> Abs/1

== system newTires/Fiala Wheel 2DOF/Fiala/Rolling/ISO ==
  "Omega " : Inport
  Fz : Inport  Port=2
  Re : Inport  Port=3
  Tamb : Inport  Port=4
  MATLAB Function : MATLAB Function  TreatAsAtomicUnit=on
  My : Outport  VectorParamsAs1DForOutWhenUnconnected=off
  wires:
  Fz/1 -> MATLAB Function/1(Fz)
  "Omega "/1 -> MATLAB Function/2(omega)
  Tamb/1 -> MATLAB Function/3(Tamb)
  Re/1 -> MATLAB Function/4(Re)
  MATLAB Function/1(My) -> My/1

== system newTires/Fiala Wheel 2DOF/Fiala/Rolling/MagicFormula ==
  "Omega " : Inport
  Fz : Inport  Port=2
  Vx : Inport  Port=3
  Fx : Inport  Port=4
  gamma : Inport  Port=5
  Prs : Inport  Port=6
  MATLAB Function : MATLAB Function  TreatAsAtomicUnit=on
  My : Outport  VectorParamsAs1DForOutWhenUnconnected=off
  wires:
  "Omega "/1 -> MATLAB Function/3(omega)
  Fz/1 -> MATLAB Function/2(Fz)
  Fx/1 -> MATLAB Function/1(Fx)
  Vx/1 -> MATLAB Function/4(Vx)
  Prs/1 -> MATLAB Function/5(press)
  gamma/1 -> MATLAB Function/6(gamma)
  MATLAB Function/1(My) -> My/1

== system newTires/Fiala Wheel 2DOF/Fiala/Rolling/Mapped ==
  "Omega " : Inport
  Fz : Inport  Port=2
  Vx : Inport  Port=3
  MATLAB Function : MATLAB Function  TreatAsAtomicUnit=on
  My : Outport  VectorParamsAs1DForOutWhenUnconnected=off
  wires:
  "Omega "/1 -> MATLAB Function/1(omega)
  Fz/1 -> MATLAB Function/2(Fz)
  Vx/1 -> MATLAB Function/3(Vx)
  MATLAB Function/1(My) -> My/1

== system newTires/Fiala Wheel 2DOF/Fiala/Rolling/None ==
  Constant2 : Constant  Value=0
  My : Outport  VectorParamsAs1DForOutWhenUnconnected=off
  wires:
  Constant2/1 -> My/1

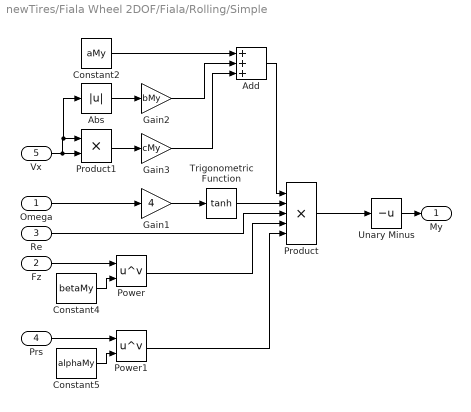
== system newTires/Fiala Wheel 2DOF/Fiala/Rolling/Simple ==
  "Omega " : Inport
  Fz : Inport  Port=2
  Re : Inport  Port=3
  Prs : Inport  Port=4
  Vx : Inport  Port=5
  Abs : Abs
  Add : Sum  Inputs=+++
  Constant2 : Constant  Value=aMy
  Constant4 : Constant  Value=betaMy
  Constant5 : Constant  Value=alphaMy
  Gain1 : Gain  Gain=4
  Gain2 : Gain  Gain=bMy
  Gain3 : Gain  Gain=cMy
  Power : Math  Operator=pow  SaturateOnIntegerOverflow=on
  Power1 : Math  Operator=pow  SaturateOnIntegerOverflow=on
  Product : Product  Inputs=5
  Product1 : Product
  Trigonometric Function : Trigonometry  Operator=tanh
  Unary Minus : UnaryMinus
  My : Outport  VectorParamsAs1DForOutWhenUnconnected=off
  wires:
  Fz/1 -> Power/1
  Gain1/1 -> Trigonometric Function/1
  Product/1 -> Unary Minus/1
  Trigonometric Function/1 -> Product/2
  "Omega "/1 -> Gain1/1
  Unary Minus/1 -> My/1
  Abs/1 -> Gain2/1
  Product1/1 -> Gain3/1
  Constant2/1 -> Add/1
  Gain2/1 -> Add/2
  Gain3/1 -> Add/3
  Re/1 -> Product/3
  Add/1 -> Product/1
  Prs/1 -> Power1/1
  Constant4/1 -> Power/2
  Constant5/1 -> Power1/2
  Power/1 -> Product/4
  Power1/1 -> Product/5
  Vx/1 -> Abs/1, Product1/1, Product1/2

== matlab function newTires/Fiala Wheel 2DOF/Fiala/Rolling/ISO/MATLAB Function ==
  data: Fz input; My output; omega input; Tamb input; Re input; Fpl parameter; Cr parameter; Kt parameter; Tmeas parameter; FZMIN parameter; FZMAX parameter; TMIN parameter; TMAX parameter
function My = ISOMy(Fz,omega,Tamb,Re,Fpl, Cr, Kt, Tmeas, FZMIN, FZMAX, TMIN, TMAX)%#codegen

coder.allowpcode('plain')
My = -automltirelongMyISO(Fz,omega,Tamb,Fpl,Cr,Kt,Tmeas,Re,FZMIN,FZMAX,TMIN,TMAX);

== matlab function newTires/Fiala Wheel 2DOF/Fiala/Rolling/MagicFormula/MATLAB Function ==
  data: Fx input; My output; Fz input; omega input; Vx input; press input; gamma input; PRESMAX parameter; FNOMIN parameter; NOMPRES parameter; QSY1 parameter; QSY2 parameter; QSY3 parameter; QSY4 parameter; QSY5 parameter; QSY6 parameter; QSY7 parameter; QSY8 parameter; lam_My parameter; UNLOADED_RADIUS parameter; FZMAX parameter; PRESMIN parameter
function My = MFMy(Fx,Fz,omega,Vx,press,gamma,PRESMAX, FNOMIN, NOMPRES, QSY1, QSY2,...%#codegen
QSY3, QSY4, QSY5, QSY6, QSY7, QSY8, lam_My, UNLOADED_RADIUS, FZMAX, PRESMIN)

My = -automltirelongMy(Fx,Fz,omega,Vx,press,FNOMIN, NOMPRES, QSY1, QSY2,...
    QSY3, QSY4,QSY5,QSY6,QSY7,QSY8,gamma,lam_My, UNLOADED_RADIUS,FZMAX,PRESMIN,PRESMAX);

== matlab function newTires/Fiala Wheel 2DOF/Fiala/Rolling/Mapped/MATLAB Function ==
  data: omega input; My output; Fz input; Vx input; VxMy parameter; FzMy parameter; MyMap parameter; FZMAX parameter
function My = MappedMy(omega,Fz,Vx,VxMy, FzMy, MyMap, FZMAX)%#codegen
coder.allowpcode('plain')
My = automltirelongMyMapped(omega,Fz,Vx,VxMy,FzMy,MyMap,FZMAX);
end
